simulink model "matlab_comm"  (R2019a)
settings: Solver=VariableStepAuto  StartTime=0.0  StopTime=inf  RelTol=1e-3
libraries: dspnetwork x2
settings Model: Creator=USRG-ASUS  LastModifiedBy=USRG-ASUS

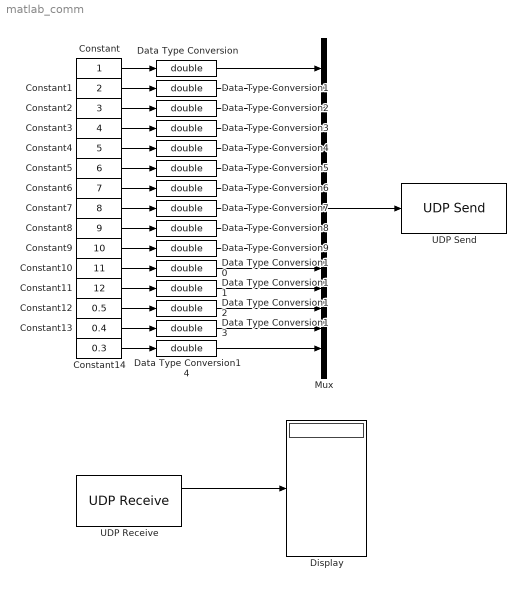
== system matlab_comm ==
  Constant : Constant
  Constant1 : Constant  Value=2
  Constant10 : Constant  Value=11
  Constant11 : Constant  Value=12
  Constant12 : Constant  Value=0.5
  Constant13 : Constant  Value=0.4
  Constant14 : Constant  Value=0.3
  Constant2 : Constant  Value=3
  Constant3 : Constant  Value=4
  Constant4 : Constant  Value=5
  Constant5 : Constant  Value=6
  Constant6 : Constant  Value=7
  Constant7 : Constant  Value=8
  Constant8 : Constant  Value=9
  Constant9 : Constant  Value=10
  Data Type Conversion{,1..14} (15 alike) : DataTypeConversion  OutDataTypeStr=double
  Display : Display
  Mux : Mux  Inputs=15
  UDP Receive : dspnetwork/UDP Receive  localURL='0.0.0.0'  localPort=9090  remoteURL='127.0.0.1'  remotePort=-1  recvBufferSize=40  dims=5  signalDatatype=double  isComplex=off  isVarSize=off  showBlockingTime=off  blockingTime=0  sampletime=-1  blockPlatform=[]
      settings: SourceProductName=Simulink
  UDP Send : dspnetwork/UDP Send  remoteURL='127.0.0.1'  remotePort=8080  localURL='0.0.0.0'  localPortSource=Automatically determine  localPort=-1  sampletime=-1  blockPlatform=[]  separateLengthPort=0
      settings: SourceProductName=Simulink
  wires:
  Mux/1 -> UDP Send/1
  UDP Receive/1 -> Display/1
  Constant/1 -> Data Type Conversion/1
  Data Type Conversion/1 -> Mux/1
  Constant1/1 -> Data Type Conversion1/1
  Data Type Conversion1/1 -> Mux/2
  Constant3/1 -> Data Type Conversion3/1
  Data Type Conversion3/1 -> Mux/4
  Constant2/1 -> Data Type Conversion2/1
  Data Type Conversion2/1 -> Mux/3
  Data Type Conversion6/1 -> Mux/7
  Data Type Conversion7/1 -> Mux/8
  Constant5/1 -> Data Type Conversion5/1
  Data Type Conversion5/1 -> Mux/6
  Constant4/1 -> Data Type Conversion4/1
  Constant7/1 -> Data Type Conversion7/1
  Constant6/1 -> Data Type Conversion6/1
  Data Type Conversion4/1 -> Mux/5
  Data Type Conversion10/1 -> Mux/11
  Data Type Conversion11/1 -> Mux/12
  Constant9/1 -> Data Type Conversion9/1
  Data Type Conversion13/1 -> Mux/14
  Data Type Conversion12/1 -> Mux/13
  Constant10/1 -> Data Type Conversion10/1
  Constant8/1 -> Data Type Conversion8/1
  Constant11/1 -> Data Type Conversion11/1
  Data Type Conversion14/1 -> Mux/15
  Constant12/1 -> Data Type Conversion12/1
  Data Type Conversion9/1 -> Mux/10
  Constant13/1 -> Data Type Conversion13/1
  Data Type Conversion8/1 -> Mux/9
  Constant14/1 -> Data Type Conversion14/1
